simulink model "AirCtl_Mon"  (R2016b)
settings: configuration reference "CodeGenConfigSet" (kept outside this file)
values from neighbouring files (symbols this model uses):
  AirCtl_dnEngTrans_C = Calibration.Parameter    [init_AirCtl_Mon.m]    (also in init_AirCtl_Mon_SIL.m = Simulink.Parameter)
  AirCtl_dqLeadTrans_C = Calibration.Parameter    [init_AirCtl_Mon.m]    (also in init_AirCtl_Mon_SIL.m = Simulink.Parameter)
  AirCtl_drAPPTrans_C = Calibration.Parameter    [init_AirCtl_Mon.m]    (also in init_AirCtl_Mon_SIL.m = Simulink.Parameter)
  AirCtl_facActDesVal_C = Calibration.Parameter    [init_AirCtl_Mon.m]    (also in init_AirCtl_Mon_SIL.m = Simulink.Parameter)
  AirCtl_facEngTempSmkHysCor_CUR = Calibration.Parameter    [init_AirCtl_Mon.m]    (also in init_AirCtl_Mon_SIL.m = Simulink.Parameter)
  AirCtl_facEngTempSmkHysCor_CURX = Calibration.Parameter    [init_AirCtl_Mon.m]    (also in init_AirCtl_Mon_SIL.m = Simulink.Parameter)
  AirCtl_facEnvPresSmkHysCor_CUR = Calibration.Parameter    [init_AirCtl_Mon.m]    (also in init_AirCtl_Mon_SIL.m = Simulink.Parameter)
  AirCtl_facEnvPresSmkHysCor_CURX = Calibration.Parameter    [init_AirCtl_Mon.m]    (also in init_AirCtl_Mon_SIL.m = Simulink.Parameter)
  AirCtl_mMaxDvt_MAP = Calibration.Parameter    [init_AirCtl_Mon.m]    (also in init_AirCtl_Mon_SIL.m = Simulink.Parameter)
  AirCtl_mMaxDvt_MAPX = Calibration.Parameter    [init_AirCtl_Mon.m]    (also in init_AirCtl_Mon_SIL.m = Simulink.Parameter)
  AirCtl_mMaxDvt_MAPY = Calibration.Parameter    [init_AirCtl_Mon.m]    (also in init_AirCtl_Mon_SIL.m = Simulink.Parameter)
  AirCtl_mMinDvt_MAP = Calibration.Parameter    [init_AirCtl_Mon.m]    (also in init_AirCtl_Mon_SIL.m = Simulink.Parameter)
  AirCtl_mMinDvt_MAPX = Calibration.Parameter    [init_AirCtl_Mon.m]    (also in init_AirCtl_Mon_SIL.m = Simulink.Parameter)
  AirCtl_mMinDvt_MAPY = Calibration.Parameter    [init_AirCtl_Mon.m]    (also in init_AirCtl_Mon_SIL.m = Simulink.Parameter)
  AirCtl_nLoIdl_C = Calibration.Parameter    [init_AirCtl_Mon.m]    (also in init_AirCtl_Mon_SIL.m = Simulink.Parameter)
  AirCtl_nOvrRun_C = Calibration.Parameter    [init_AirCtl_Mon.m]    (also in init_AirCtl_Mon_SIL.m = Simulink.Parameter)
  AirCtl_numAirTempMon_C = Calibration.Parameter    [init_AirCtl_Mon.m]    (also in init_AirCtl_Mon_SIL.m = Simulink.Parameter)
  AirCtl_numEngTempMon_C = Calibration.Parameter    [init_AirCtl_Mon.m]    (also in init_AirCtl_Mon_SIL.m = Simulink.Parameter)
  AirCtl_pAirHi_C = Calibration.Parameter    [init_AirCtl_Mon.m]    (also in init_AirCtl_Mon_SIL.m = Simulink.Parameter)
  AirCtl_pAirLo_C = Calibration.Parameter    [init_AirCtl_Mon.m]    (also in init_AirCtl_Mon_SIL.m = Simulink.Parameter)
  AirCtl_qEngTempSmkHysCor_MAP = Calibration.Parameter    [init_AirCtl_Mon.m]    (also in init_AirCtl_Mon_SIL.m = Simulink.Parameter)
  AirCtl_qEngTempSmkHysCor_MAPX = Calibration.Parameter    [init_AirCtl_Mon.m]    (also in init_AirCtl_Mon_SIL.m = Simulink.Parameter)
  AirCtl_qEngTempSmkHysCor_MAPY = Calibration.Parameter    [init_AirCtl_Mon.m]    (also in init_AirCtl_Mon_SIL.m = Simulink.Parameter)
  AirCtl_qEnvPresSmkHysCor_MAP = Calibration.Parameter    [init_AirCtl_Mon.m]    (also in init_AirCtl_Mon_SIL.m = Simulink.Parameter)
  AirCtl_qEnvPresSmkHysCor_MAPX = Calibration.Parameter    [init_AirCtl_Mon.m]    (also in init_AirCtl_Mon_SIL.m = Simulink.Parameter)
  AirCtl_qEnvPresSmkHysCor_MAPY = Calibration.Parameter    [init_AirCtl_Mon.m]    (also in init_AirCtl_Mon_SIL.m = Simulink.Parameter)
  AirCtl_qOvrRun_C = Calibration.Parameter    [init_AirCtl_Mon.m]    (also in init_AirCtl_Mon_SIL.m = Simulink.Parameter)
  AirCtl_qSmkHys_MAP = Calibration.Parameter    [init_AirCtl_Mon.m]    (also in init_AirCtl_Mon_SIL.m = Simulink.Parameter)
  AirCtl_qSmkHys_MAPX = Calibration.Parameter    [init_AirCtl_Mon.m]    (also in init_AirCtl_Mon_SIL.m = Simulink.Parameter)
  AirCtl_qSmkHys_MAPY = Calibration.Parameter    [init_AirCtl_Mon.m]    (also in init_AirCtl_Mon_SIL.m = Simulink.Parameter)
  AirCtl_qSwtSmkHi_C = Calibration.Parameter    [init_AirCtl_Mon.m]    (also in init_AirCtl_Mon_SIL.m = Simulink.Parameter)
  AirCtl_qSwtSmkLo_C = Calibration.Parameter    [init_AirCtl_Mon.m]    (also in init_AirCtl_Mon_SIL.m = Simulink.Parameter)
  AirCtl_rEGRDflVal_CA = Calibration.Parameter    [init_AirCtl_Mon.m]    (also in init_AirCtl_Mon_SIL.m = Simulink.Parameter)
  AirCtl_rTVADflVal_CA = Calibration.Parameter    [init_AirCtl_Mon.m]    (also in init_AirCtl_Mon_SIL.m = Simulink.Parameter)
  AirCtl_stPrioMon_CA = Calibration.Parameter    [init_AirCtl_Mon.m]    (also in init_AirCtl_Mon_SIL.m = Simulink.Parameter)
  AirCtl_swtGovDvtMonEna_C = Calibration.Parameter    [init_AirCtl_Mon.m]    (also in init_AirCtl_Mon_SIL.m = Simulink.Parameter)
  AirCtl_tAirCldHi_C = Calibration.Parameter    [init_AirCtl_Mon.m]    (also in init_AirCtl_Mon_SIL.m = Simulink.Parameter)
  AirCtl_tAirCldLo_C = Calibration.Parameter    [init_AirCtl_Mon.m]    (also in init_AirCtl_Mon_SIL.m = Simulink.Parameter)
  AirCtl_tAirWrmHi_C = Calibration.Parameter    [init_AirCtl_Mon.m]    (also in init_AirCtl_Mon_SIL.m = Simulink.Parameter)
  AirCtl_tAirWrmLo_C = Calibration.Parameter    [init_AirCtl_Mon.m]    (also in init_AirCtl_Mon_SIL.m = Simulink.Parameter)
  AirCtl_tClntCldHi_C = Calibration.Parameter    [init_AirCtl_Mon.m]    (also in init_AirCtl_Mon_SIL.m = Simulink.Parameter)
  AirCtl_tClntCldLo_C = Calibration.Parameter    [init_AirCtl_Mon.m]    (also in init_AirCtl_Mon_SIL.m = Simulink.Parameter)
  AirCtl_tClntWrmHi_C = Calibration.Parameter    [init_AirCtl_Mon.m]    (also in init_AirCtl_Mon_SIL.m = Simulink.Parameter)
  AirCtl_tClntWrmLo_C = Calibration.Parameter    [init_AirCtl_Mon.m]    (also in init_AirCtl_Mon_SIL.m = Simulink.Parameter)
  AirCtl_tiCldStrt_CUR = Calibration.Parameter    [init_AirCtl_Mon.m]    (also in init_AirCtl_Mon_SIL.m = Simulink.Parameter)
  AirCtl_tiCldStrt_CURX = Calibration.Parameter    [init_AirCtl_Mon.m]    (also in init_AirCtl_Mon_SIL.m = Simulink.Parameter)
  AirCtl_tiClth_C = Calibration.Parameter    [init_AirCtl_Mon.m]    (also in init_AirCtl_Mon_SIL.m = Simulink.Parameter)
  AirCtl_tiDynSmkDly_C = Calibration.Parameter    [init_AirCtl_Mon.m]    (also in init_AirCtl_Mon_SIL.m = Simulink.Parameter)
  AirCtl_tiGovDvtMaxDebDef_C = Calibration.Parameter    [init_AirCtl_Mon.m]    (also in init_AirCtl_Mon_SIL.m = Simulink.Parameter)
  AirCtl_tiGovDvtMaxDebOk_C = Calibration.Parameter    [init_AirCtl_Mon.m]    (also in init_AirCtl_Mon_SIL.m = Simulink.Parameter)
  AirCtl_tiGovDvtMinDebDef_C = Calibration.Parameter    [init_AirCtl_Mon.m]    (also in init_AirCtl_Mon_SIL.m = Simulink.Parameter)
  AirCtl_tiGovDvtMinDebOk_C = Calibration.Parameter    [init_AirCtl_Mon.m]    (also in init_AirCtl_Mon_SIL.m = Simulink.Parameter)
  AirCtl_tiLoIdl_C = Calibration.Parameter    [init_AirCtl_Mon.m]    (also in init_AirCtl_Mon_SIL.m = Simulink.Parameter)
  AirCtl_tiStatSmkDly_C = Calibration.Parameter    [init_AirCtl_Mon.m]    (also in init_AirCtl_Mon_SIL.m = Simulink.Parameter)
  AirCtl_tiTransDly_C = Calibration.Parameter    [init_AirCtl_Mon.m]    (also in init_AirCtl_Mon_SIL.m = Simulink.Parameter)
  AirCtl_uBattThres_C = Calibration.Parameter    [init_AirCtl_Mon.m]    (also in init_AirCtl_Mon_SIL.m = Simulink.Parameter)
  ASMod_numBnk_C = Calibration.Parameter    [init_AirCtl_Mon.m]    (also in init_AirCtl_Mon_SIL.m = Simulink.Parameter)
  Epm_numCyl_C = Calibration.Parameter    [init_AirCtl_Mon.m]    (also in init_AirCtl_Mon_SIL.m = Simulink.Parameter)
undefined symbols (not defined in the file or in its folder): AirCtl_Mon_DT, EngState_conv, Switch_conv
libraries: simulink x45, CXLib x23
(part 1 of 4)
settings Model: Creator=Wollf  LastModifiedBy=guanxiaoxing
settings ConfigSetRef: SourceLocation=Base Workspace

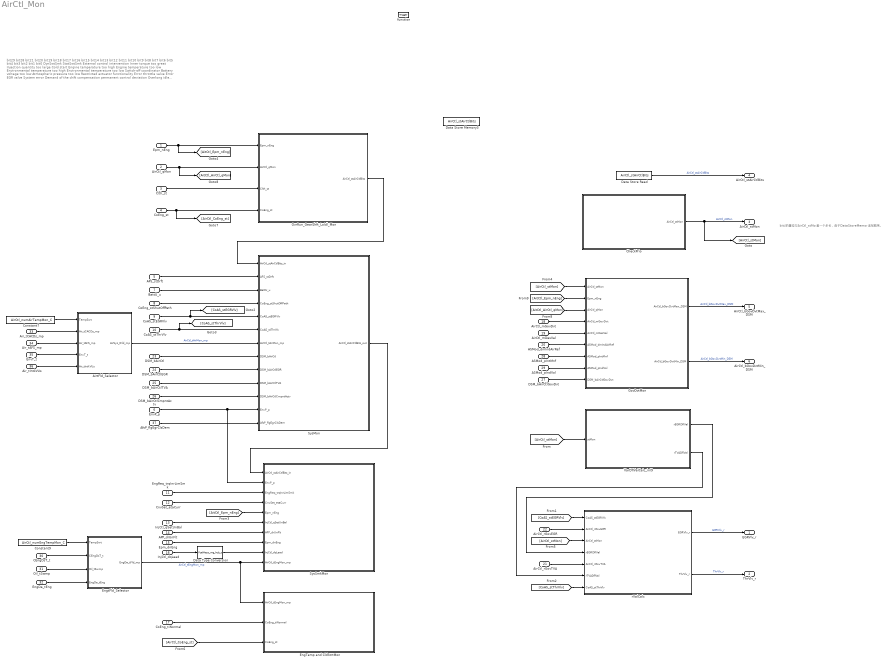
== system AirCtl_Mon ==
  note: bit4的置位与AirCtl_stMon差一个步长，由于DataStoreMemory读写顺序。
  note: bit29
      | bit28
      | bit21
      | bit20
      | bit19
      | bit18
      | bit17
      | bit16
      | bit15
      | bit14
      | bit13
      | bit12
      | bit11
      | bit10
      | bit9
      | bit8
      | bit7
      | bit6
      | bit5
      | bit4
      | bit3
      | bit2
      | bit1
      | bit0
      |
      | DynSwtSmk
      | StatSwtSmk
      | External control intervention
      | Inner torque too great
      |
      | Injection quantity too
      | large
      | Cold start
      | Engine temperature
      | too high
      | Engine temperature
      | too low
      | Environmental temperature too high
      | Environmental temperature too low
      | Switch-off coordinator
      | Battery voltage too
      | low
      | Atmospheric pressure
      | too low
      | Restricted
      | actuator functionality
      | Error throttle valve
      | Error EGR valve
      | System error
      | Demand of
      | the drift
      | compensation
      | permanent control
      | deviation
      | Overlong
      | idle
      | Gear shifting
      | Overrun
      | Normal
      | operation
      |
      | 使用动态冒烟限制
      | 使用静态冒烟限制
      | 外部控制
      | 内部扭矩太大
      |
      | 喷油量太大
      | 处在启动的工况
      | 发动机温度太高
      | 发动机温度太低
      | 环境温度太高
      | 环境温度太低
      | 开关关闭
      | 蓄电池电压过低
      | 大气压力过低
      | 执行器功能被限制
      | 节气门阀故障
      | EGR阀故障
      | 系统故障
      | 零点漂移补偿
      | 存在控制偏差
      | 长时间怠速状态
      | 换挡情况
      | 超速工况
      | 正常模式
  Epm_nEng : Inport  Tag=rpm  Description=Engine speed  OutMin=0  OutMax=6000  OutDataTypeStr=EngSpeed_rpm
  AirCtl_qMon : Inport  Tag=mg/hub  Description=Inner quantity of monitoring level for open-loop control of the exhaustgas recirculation control  Port=2  OutMin=-319  OutMax=319  OutDataTypeStr=FuelMass_mg_hub
  Clth_st : Inport  Description=Clutch information  Port=3  OutMin=0  OutMax=255  OutDataTypeStr=State_uint8
  CoEng_st : Inport  Description=Engine coordinator state  Port=4  OutDataTypeStr=Enum: EngState_conv
  AFS_stDrft : Inport  Description=Status of drift compensation  Port=5  OutMin=0  OutMax=255  OutDataTypeStr=State_uint8
  EnvP_p : Inport  Tag=kPa  Description=Barometric pressure  Port=6  OutMin=0  OutMax=3276  OutDataTypeStr=AirPressure_kPa
  BattU_u : Inport  Tag=mv  Description=Battery voltage  Port=7  OutMin=0  OutMax=50000  OutDataTypeStr=Battery_mv
  CoEng_stShutOffPath : Inport  Description=Active shut-off paths resulting from active reversible,irreversible and afterrun shut-off paths  Port=8  OutMin=0  OutMax=65535  OutDataTypeStr=State_uint16
  CoAS_stEGRVlv : Inport  Description="State  of EGR control enable"  Port=9  OutMin=0  OutMax=255  OutDataTypeStr=State_uint8
  CoAS_stThrVlv : Inport  Description="State  of TVA control enable"  Port=10  OutMin=0  OutMax=255  OutDataTypeStr=State_uint8
  EngReq_trqInrLimSmk : Inport  Tag=Nm  Description=Limiting torque smoke limit  Port=11  OutMin=-3276.8  OutMax=3276.7  OutDataTypeStr=Trq_Nm
  CnvSet_etaCurr : Inport  Tag=Nm/(mg/hub)  Description=Current conversion efficiency  Port=12  OutMin=-255  OutMax=255  OutDataTypeStr=TrqEta_Nm_mg_hub
  InjCtl_qSetUnBal : Inport  Tag=mg/hub  Description=Current injection quantity  Port=13  OutMin=-319  OutMax=319  OutDataTypeStr=FuelMass_mg_hub
  APP_drUnFlt : Inport  Tag=%/s  Description=Acceleration pedal position gradient of unfilterd value  Port=14  OutMin=-100000  OutMax=100000  OutDataTypeStr=Accpedal_rate_s
  Epm_dnEng : Inport  Tag=rpm/s  Description=Engine speed gradient calculated over current crankshaft-segment (S0-S0 or S1-S1)  Port=15  OutMin=-12000  OutMax=12000  OutDataTypeStr=EngSpeed_rpm_s
  InjCtl_dqLead : Inport  Tag=mg/hub  Description=Gradient of quantity  Port=16  OutMin=-319  OutMax=319  OutDataTypeStr=FuelMass_mg_hub
  CoEng_tiNormal : Inport  Tag=ms  Description="Time since state\"CONENG_RUNNING\"was reached"  Port=17  OutMin=0  OutMax=42949672950  OutDataTypeStr=EngTime_ms
  AirCtl_mGovDvt : Inport  Tag=mg/hub  Description=Deviation of Air mass  Port=18  OutMin=-15000  OutMax=15000  OutDataTypeStr=AirMass_mg_hub
  AirCtl_mDesVal : Inport  Tag=mg/hub  Description=Desired air mass  Port=19  OutMin=-15000  OutMax=15000  OutDataTypeStr=AirMass_mg_hub
  ASMod_dmIndAirRef : Inport  Tag=kg/h  Description=Reference of gas mass flow into the engine while exhaust-gas recirculation is closed  Port=20  OutMin=-8192  OutMax=8191  OutDataTypeStr=AirMassPerTime
  AirCtl_rGovTVA : Inport  Tag=%  Description=Opening for intake throttle (TVA)  Port=21  OutMin=-100  OutMax=100  OutDataTypeStr=Prc_100_rate
  AirCtl_rGovEGR : Inport  Tag=%  Description=Setpoint position of the exhaust-gas recirculation valve from the exhaust-gas recirculation control  Port=22  OutMin=-100  OutMax=100  OutDataTypeStr=Prc_100_rate
  DSM_bAirCtl : Inport  Description=Status of Fid_AirCtl  Port=23  OutMin=0  OutMax=1  OutDataTypeStr=boolean
  DSM_bAirCtlEGR : Inport  Description=Status of Fid_AirCtlEGR  Port=24  OutMin=0  OutMax=1  OutDataTypeStr=boolean
  DSM_bAirCtlTVA : Inport  Description=Status of Fid_AirCtlTVA  Port=25  OutMin=0  OutMax=1  OutDataTypeStr=boolean
  DSM_bAirCtlCmpntActv : Inport  Description=Status of Fid_AirCtlCmpntActv  Port=26  OutMin=0  OutMax=1  OutDataTypeStr=boolean
  DSM_bAirCtlGovDvt : Inport  Description=Status of Fid_AirCtlGovDvt  Port=27  OutMin=0  OutMax=1  OutDataTypeStr=boolean
  ASMod_pIntMnf : Inport  Tag=kPa  Description=Pressure in the intake manifold  Port=28  OutMin=0  OutMax=3000  OutDataTypeStr=AirPressure_kPa
  ASMod_pIndVol : Inport  Tag=kPa  Description=Pressure in the induction volume  Port=29  OutMin=0  OutMax=3000  OutDataTypeStr=AirPressure_kPa
  CEngDsT_t : Inport  Tag=deg  Description=engine coolant temperature after filter  Port=30  OutMin=-200  OutMax=200  OutDataTypeStr=Temp_deg
  Oil_tSwmp : Inport  Tag=deg  Description=Oil temperature in oil sump  Port=31  OutMin=-50  OutMax=200  OutDataTypeStr=Temp_deg
  EngDa_tEng : Inport  Tag=deg  Description=Engine temperature  Port=32  OutMin=-1000  OutMax=1000  OutDataTypeStr=Temp_deg
  Air_tCACDs_mp : Inport  Tag=deg  Description=Charge-air temperature downstream from charge-air cooler  Port=33  OutMin=-200  OutMax=200  OutDataTypeStr=Temp_deg
  Air_tAFS_mp : Inport  Tag=deg  Description=Induction air temperature at the HFM  Port=34  OutMin=-200  OutMax=200  OutDataTypeStr=Temp_deg
  EnvT_t : Inport  Tag=deg  Description=Environmental temperature  Port=35  OutMin=-200  OutMax=200  OutDataTypeStr=Temp_deg
  Air_tIntkVUs : Inport  Tag=deg  Description=Intake air temperature upstream of the inlet valve  Port=36  OutMin=-200  OutMax=200  OutDataTypeStr=Temp_deg
  AfsP_flgEgrClsDem : Inport  Description=Flag to indicate the requirement of a shutoff case for closing the EGR valve  Port=37  OutMin=0  OutMax=1  OutDataTypeStr=boolean
  function : TriggerPort  TriggerType=function-call  VariantControl=Variant
  AirtFld_Selector : Subsystem
  CheckPrio : Subsystem
  Constant7 : Constant  Value=AirCtl_numAirTempMon_C
  Constant9 : Constant  Value=AirCtl_numEngTempMon_C
  Data Store Memory3 : DataStoreMemory  DataStoreName=AirCtl_stAirCtlBits  ReadBeforeWriteMsg=warning  WriteAfterWriteMsg=warning  WriteAfterReadMsg=warning  ShowAdditionalParam=off  OutDataTypeStr=uint32
  Data Store Read : DataStoreRead  DataStoreName=AirCtl_stAirCtlBits
  Data Type Conversion : DataTypeConversion  OutDataTypeStr=FuelMass_mg_hub_s
  EngTemp and CldStrtMon : Subsystem
  EngtFld_Selector : Subsystem
  GovDvtMon : Subsystem
  OvrRun_GearShft_LoIdl_Mon : Subsystem
  SysMon : Subsystem
  SysSmkMon : Subsystem
  VarDflValCalc_inl9 : Subsystem
  rValCalc : Subsystem
  EGRVlv_r : Outport  Tag=%  Description=Commanded value from application SW  OutMin=-100  OutMax=100  OutDataTypeStr=Prc_100_rate
  ThrVlv_r : Outport  Tag=%  Description=Commanded value from application SW  Port=2  OutMin=-100  OutMax=100  OutDataTypeStr=Prc_100_rate
  AirCtl_stMon : Outport  Description=status: shutdown case of the governor  Port=3  OutMin=0  OutMax=255  OutDataTypeStr=State_uint8
  AirCtl_stAirCtlBits : Outport  Description=Status of the switch-off events of the exhaust-gas recirculation control, monitoring  Port=4  OutMin=0  OutMax=4294967295  OutDataTypeStr=State_uint32
  AirCtl_bGovDvtMax_DSM : Outport  Description=DFC of AirCtl_bGovDvtMax  Port=5  OutMin=0  OutMax=1  OutDataTypeStr=boolean
  AirCtl_bGovDvtMin_DSM : Outport  Description=DFC of AirCtl_bGovDvtMin  Port=6  OutMin=0  OutMax=1  OutDataTypeStr=boolean
  wires:
  CheckPrio/1(AirCtl_stMon) -> AirCtl_stMon/1, [AirCtl_stMon]  "AirCtl_stMon"
  Data Store Read/1 -> AirCtl_stAirCtlBits/1  "AirCtl_stAirCtlBits"
  GovDvtMon/1(AirCtl_bGovDvtMax_DSM) -> AirCtl_bGovDvtMax_DSM/1  "AirCtl_bGovDvtMax_DSM"
  GovDvtMon/2(AirCtl_bGovDvtMin_DSM) -> AirCtl_bGovDvtMin_DSM/1  "AirCtl_bGovDvtMin_DSM"
  CnvSet_etaCurr/1 -> SysSmkMon/4(CnvSet_etaCurr)
  SysMon/1(AirCtl_stAirCtlBits_out) -> SysSmkMon/1(AirCtl_stAirCtlBits_in)
  OvrRun_GearShft_LoIdl_Mon/1(AirCtl_stAirCtlBits) -> SysMon/1(AirCtl_stAirCtlBits_in)
  EngtFld_Selector/1(EngDa_tFld_mp) -> EngTemp and CldStrtMon/1(AirCtl_tEngMon_mp), SysSmkMon/10(AirCtl_tEngMon_mp)  "AirCtl_tEngMon_mp"
  AirtFld_Selector/1(AirSys_tFld_mp) -> SysMon/7(" AirCtl_tAirMon_mp")  "AirCtl_tAirMon_mp"
  ASMod_pIndVol/1 -> GovDvtMon/8(ASMod_pIndVol)
  AirCtl_mDesVal/1 -> GovDvtMon/5(AirCtl_mDesVal)
  ASMod_pIntMnf/1 -> GovDvtMon/7(ASMod_pIntMnf)
  ASMod_dmIndAirRef/1 -> GovDvtMon/6(ASMod_dmIndAirRef)
  AirCtl_qMon/1 -> OvrRun_GearShft_LoIdl_Mon/2(AirCtl_qMon), [AitCtl_AirCtl_qMon]
  Epm_nEng/1 -> OvrRun_GearShft_LoIdl_Mon/1(Epm_nEng), [AitCtl_Epm_nEng]
  CoEng_st/1 -> OvrRun_GearShft_LoIdl_Mon/4(CoEng_st), [AirCtl_CoEng_st]
  AirCtl_mGovDvt/1 -> GovDvtMon/4(AirCtl_mGovDvt)
  Clth_st/1 -> OvrRun_GearShft_LoIdl_Mon/3(Clth_st)
  CoAS_stThrVlv/1 -> [CoAS_stThrVlv], SysMon/6(CoAS_stThrVlv)
  CoEng_stShutOffPath/1 -> SysMon/4(CoEng_stShutOffPath)
  AFS_stDrft/1 -> SysMon/2(AFS_stDrft)
  [AitCtl_Epm_nEng] -> GovDvtMon/2(Epm_nEng)
  EnvP_p/1 -> SysSmkMon/2(EnvP_p), SysMon/12(EnvP_p)
  EngReq_trqInrLimSmk/1 -> SysSmkMon/3(EngReq_trqInrLimSmk)
  [AirCtl_CoEng_st] -> EngTemp and CldStrtMon/3(CoEng_st)
  BattU_u/1 -> SysMon/3(BattU_u)
  CoAS_stEGRVlv/1 -> [CoAS_stEGRVlv], SysMon/5(CoAS_stEGRVlv)
  [AitCtl_Epm_nEng] -> SysSmkMon/5(Epm_nEng)
  InjCtl_qSetUnBal/1 -> SysSmkMon/6(InjCtl_qSetUnBal)
  InjCtl_dqLead/1 -> Data Type Conversion/1
  CoEng_tiNormal/1 -> EngTemp and CldStrtMon/2(CoEng_tiNormal)
  APP_drUnFlt/1 -> SysSmkMon/7(APP_drUnFlt)
  [AitCtl_AirCtl_qMon] -> GovDvtMon/3(AirCtl_qMon)
  Epm_dnEng/1 -> SysSmkMon/8(Epm_dnEng)
  DSM_bAirCtl/1 -> SysMon/8(DSM_bAirCtl)
  DSM_bAirCtlEGR/1 -> SysMon/9(DSM_bAirCtlEGR)
  DSM_bAirCtlTVA/1 -> SysMon/10(DSM_bAirCtlTVA)
  DSM_bAirCtlCmpntActv/1 -> SysMon/11(DSM_bAirCtlCmpntActv)
  [CoAS_stEGRVlv] -> rValCalc/1(CoAS_stEGRVlv)
  AirCtl_rGovEGR/1 -> rValCalc/2(AirCtl_rGovEGR)
  VarDflValCalc_inl9/1(rEGRDflVal) -> rValCalc/4(rEGRDflVal)
  AirCtl_rGovTVA/1 -> rValCalc/5(AirCtl_rGovTVA)
  VarDflValCalc_inl9/2(rTVADflVal) -> rValCalc/6(rTVADflVal)
  [CoAS_stThrVlv] -> rValCalc/7(CoAS_stThrVlv)
  rValCalc/1(EGRVlv_r) -> EGRVlv_r/1  "EGRVlv_r"
  rValCalc/2(ThrVlv_r) -> ThrVlv_r/1  "ThrVlv_r"
  [AirCtl_stMon] -> VarDflValCalc_inl9/1(stMon)
  [AirCtl_stMon] -> GovDvtMon/1(AirCtl_stMon)
  [AirCtl_stMon] -> rValCalc/3(AirCtl_stMon)
  DSM_bAirCtlGovDvt/1 -> GovDvtMon/9(DSM_bAirCtlGovDvt)
  CEngDsT_t/1 -> EngtFld_Selector/2(CEngDsT_t)
  Oil_tSwmp/1 -> EngtFld_Selector/3(Oil_tSwmp)
  EngDa_tEng/1 -> EngtFld_Selector/4(EngDa_tEng)
  Air_tAFS_mp/1 -> AirtFld_Selector/3(Air_tAFS_mp)
  Air_tCACDs_mp/1 -> AirtFld_Selector/2(Air_tCACDs_mp)
  EnvT_t/1 -> AirtFld_Selector/4(EnvT_t)
  Air_tIntkVUs/1 -> AirtFld_Selector/5(Air_tIntkVUs)
  Constant7/1 -> AirtFld_Selector/1(TempSwt)
  Constant9/1 -> EngtFld_Selector/1(TempSwt)
  Data Type Conversion/1 -> SysSmkMon/9(InjCtl_dqLead)
  AfsP_flgEgrClsDem/1 -> SysMon/13(AfsP_flgEgrClsDem)

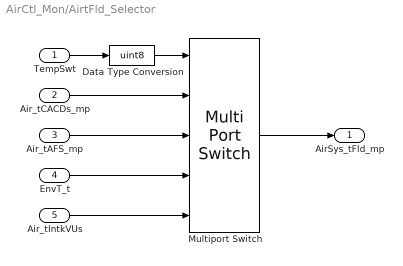
== system AirCtl_Mon/AirtFld_Selector ==
  TempSwt : Inport
  Air_tCACDs_mp : Inport  Tag=deg  Description=Charge-air temperature downstream from charge-air cooler  Port=2
  Air_tAFS_mp : Inport  Tag=deg  Description=Induction air temperature at the HFM  Port=3
  EnvT_t : Inport  Tag=deg  Description=Environmental temperature  Port=4
  Air_tIntkVUs : Inport  Tag=deg  Description=Intake air temperature upstream of the inlet valve  Port=5
  Data Type Conversion : DataTypeConversion  OutDataTypeStr=uint8
  Multiport Switch : MultiPortSwitch  DataPortOrder=Zero-based contiguous  Inputs=4
  AirSys_tFld_mp : Outport  Tag=deg  Description=Engine temperature field
  wires:
  Air_tCACDs_mp/1 -> Multiport Switch/2
  Multiport Switch/1 -> AirSys_tFld_mp/1
  EnvT_t/1 -> Multiport Switch/4
  Air_tAFS_mp/1 -> Multiport Switch/3
  Data Type Conversion/1 -> Multiport Switch/1
  TempSwt/1 -> Data Type Conversion/1
  Air_tIntkVUs/1 -> Multiport Switch/5
